simulink model "UDPTest_backup"  (R2024b)
settings: Solver=FixedStepAuto  StartTime=0.0  StopTime=Inf  FixedStep=.001  RelTol=1e-3
libraries: slrealtimeiplib x5, etargetslib x2
settings Model: PacingRate=25  Creator=operator  LastModifiedBy=santh
settings RTWCC: GPUComputeCapability=3.5

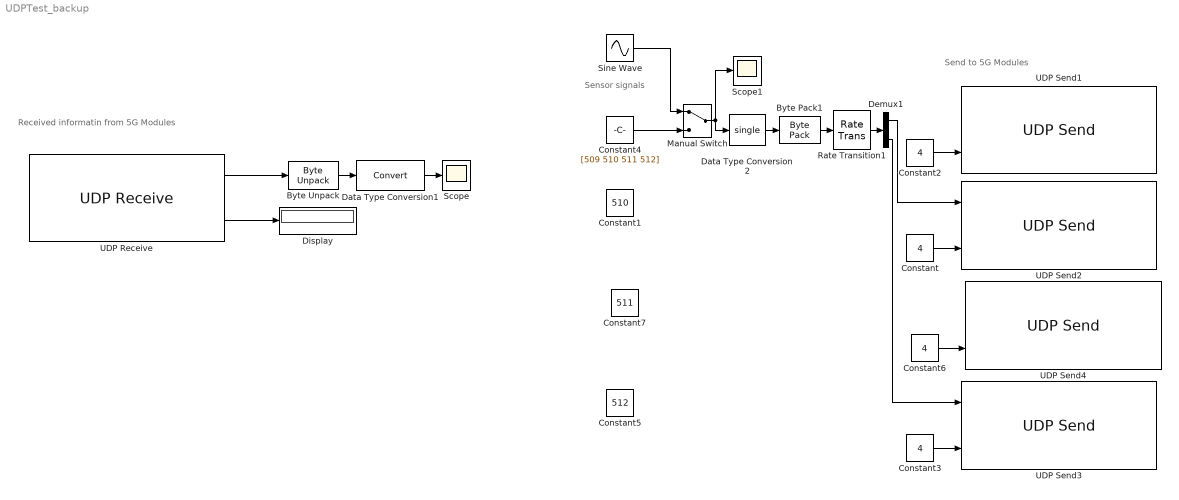
== system UDPTest_backup ==
  note: Sensor signals
  note: Send to 5G Modules
  note: Received informatin from 5G Modules
  Byte Pack1 : etargetslib/Byte Pack  datatypes={'single'}  byteAlign=1
  Byte Unpack : etargetslib/Byte Unpack  dimensions={[1]}  datatypes={'single'}  byteAlign=1
  Constant{,2..3,6} (4 alike) : Constant  Value=4  SampleTime=1
  Constant1 : Constant  Value=510  SampleTime=1
  Constant4 : Constant  Value=[509 510 511 512]  SampleTime=-1
  Constant5 : Constant  Value=512  SampleTime=-1
  Constant7 : Constant  Value=511  SampleTime=-1
  Data Type Conversion1 : DataTypeConversion  SaturateOnIntegerOverflow=off  RndMeth=Floor
  Data Type Conversion2 : DataTypeConversion  OutDataTypeStr=single  SaturateOnIntegerOverflow=off  RndMeth=Floor
  Demux1 : Demux  Outputs=2
  Display : Display
  Manual Switch : ManualSwitch
  Rate Transition1 : RateTransition  OutPortSampleTime=1
  Scope : Scope
  Scope1 : Scope
  Sine Wave : Sin  Amplitude=[110 110 110 20]  Frequency=50*2*3.1415926  Phase=[0 2*pi/3 4*pi/3 0]  SampleTime=0
  UDP Receive : slrealtimeiplib/UDP Receive  useHostTargetConn=off  ipAddress=172.16.11.69  localPort=8080  rcvWidth=4  rcvFmAny=on  fmAddress=172.16.11.21  sampleTime=-1  enableMessage=off  maxPackets=1
  UDP Send1 : slrealtimeiplib/UDP Send  useHostTargetConn=off  toAddress=172.16.11.9  toPort=7000  sampleTime=1  enableMessage=off  ipAddress=172.16.11.69  localPort=5005
  UDP Send2 : slrealtimeiplib/UDP Send  useHostTargetConn=off  toAddress=172.16.11.10  toPort=7000  sampleTime=1  enableMessage=off  ipAddress=172.16.11.69  localPort=5005
  UDP Send3 : slrealtimeiplib/UDP Send  useHostTargetConn=off  toAddress=172.16.11.12  toPort=7000  sampleTime=1  enableMessage=off  ipAddress=172.16.11.69  localPort=5005
  UDP Send4 : slrealtimeiplib/UDP Send  useHostTargetConn=off  toAddress=172.16.11.11  toPort=7000  sampleTime=1  enableMessage=off  ipAddress=172.16.11.69  localPort=5005
  wires:
  Data Type Conversion2/1 -> Byte Pack1/1
  UDP Receive/2 -> Display/1
  UDP Receive/1 -> Byte Unpack/1
  Byte Unpack/1 -> Data Type Conversion1/1
  Byte Pack1/1 -> Rate Transition1/1
  Rate Transition1/1 -> Demux1/1
  Data Type Conversion1/1 -> Scope/1
  Constant2/1 -> UDP Send1/2
  Constant3/1 -> UDP Send3/2
  Constant/1 -> UDP Send2/2
  Constant6/1 -> UDP Send4/2
  Sine Wave/1 -> Manual Switch/1
  Constant4/1 -> Manual Switch/2
  Manual Switch/1 -> Data Type Conversion2/1, Scope1/1
  Demux1/1 -> UDP Send2/1
  Demux1/2 -> UDP Send3/1
